simulink model "wheel_leg"  (R2025b)
settings: Solver=VariableStepAuto  StartTime=0.0  StopTime=10  FixedStep=0.0001  RelTol=1e-3
values from neighbouring files (symbols this model uses):
  g = 9.8    [part1_dynamic.m]    (also in simulation.m)
  M_L_support = 1.44/2 + 0.045*2    (= 0.81)    [part1_dynamic.m]
  N = length(x_uniform)    [sweep_Ncut.m]
  N_filter = results(i).N    [sweep_Ncut.m]
  X = [theta; dtheta; x; dx; phi; dphi]    [part1_dynamic.m]    (also in simulation.m)
  Y = fft(x_uniform)    [sweep_Ncut.m]
undefined symbols (not defined in the file or in its folder): KD_leg, KP_leg, Z
libraries: sm_lib x76, nesl_utility x20, slpidlib x4
(part 1 of 3)
settings Model: PauseTimes=10  Creator=Hhop  LastModifiedBy=13422
settings SolverCC: AlgebraicLoopSolver=TrustRegion  MinimalZcImpactIntegration=on
settings DebuggingCC: ReadBeforeWriteMsg=DisableAll  WriteAfterWriteMsg=DisableAll  WriteAfterReadMsg=DisableAll  MultiTaskDSMMsg=none
settings ModelReferenceCC: UpdateModelReferenceTargets=IfOutOfDate
settings SFSimCC: SFSimEcho=off
settings RTWCC: GPUComputeCapability=3.5  DLArmComputeVersion=19.05

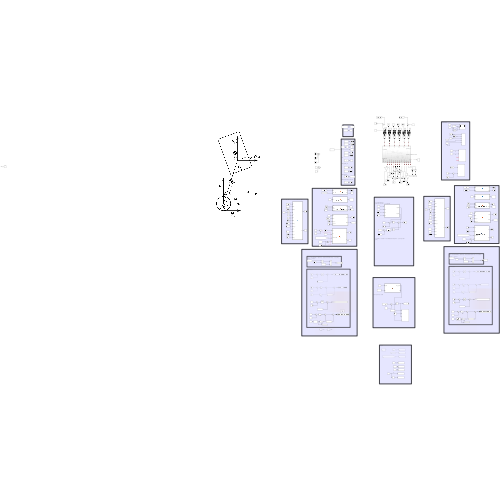
[thumbnail: Simulink's stored preview of the top-level diagram]
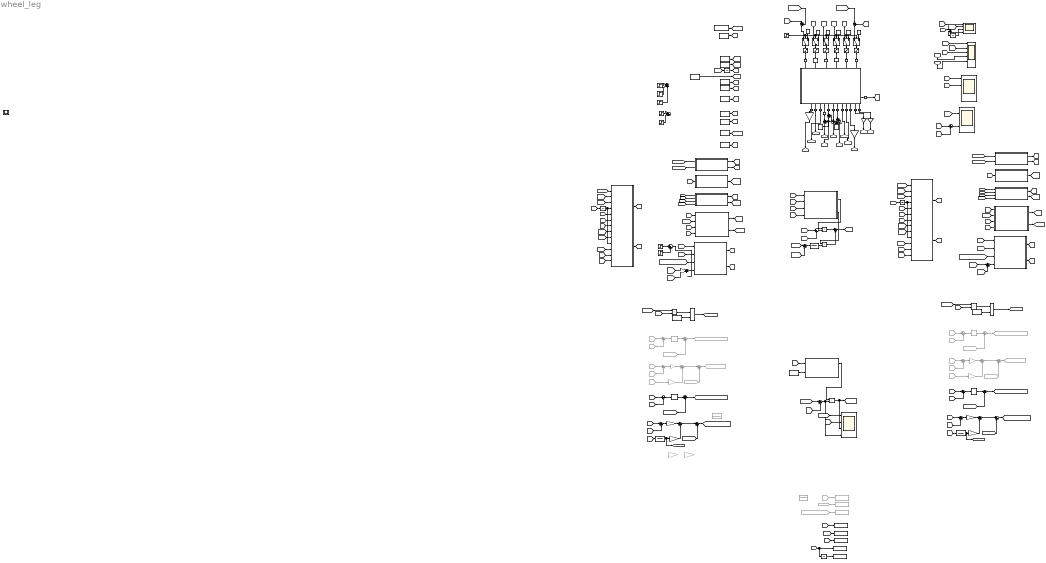
== system wheel_leg ==
  note: 转向控制器
      |
      |
      |
      |
      |
      |
      |
      |
      |
      |
      |
      |
      |
      |
      |
      |
      | 注意从左向右转是正方向啊
  note: 抑制劈叉控制器
      |
      |
      |
      |
      | 这个是等效摆的弹簧阻尼
      | 这个腾空依旧可以控制住，这个是慢控制器
      |
      |
      |
      |
      |
      |
      |
      |
      |
      |
      |
      |
      |
      |
      |
      |
      |
      |
      |
      |
      |
      |
      |
      |
      |
      |
      |
      |
      |
      |
      |
      |
      |
      |
      |
      | 这个是加到轮子上的控制器，在轮子解除地面的时候快速相应，这个是快速控制器
      | (这个和)
  note: 数据实时观测
  note: 数据打印
  note: 整个单边支持力的输出
  note: 腿长保持控制器
  note: 计算单腿支持力前馈，先只用前馈加上去，开环。之后再闭环.
      | 另外，先不除以costheta了，数值不稳定，而且线性化就是大概在1附近。为了更加稳定
      | 直接除以一个衰减因子
  note: X_d
      |
      |
      |
      |
      |
      |
      |
      |
      |
      |
      |
      |
      |
      |
      |
      |
      |
      |
      | L0d
      |
      |
      |
      |
      |
      | pai0_Diff_PD_ctrl
      |
      |
      |
      |
      |
      |
      |
      |
      |
      |
      | yaw轴速度目标
      |
      |
      |
      |
      | yaw轴速度控制器相应速度参数
  note: 这里面dx与x默认RL一样了，之后考虑不对称的时候在改
  note: 整个单边支持力的输出
  note: 腿长保持控制器
  note: 计算单腿支持力前馈，先只用前馈加上去，开环。之后再闭环.
      | 另外，先不除以costheta了，数值不稳定，而且线性化就是大概在1附近。为了更加稳定
      | 直接除以一个衰减因子
  note: 这里面dx与x默认RL一样了，之后考虑不对称的时候在改
  Constant : Constant  Value=M_L_support
  Constant1 : Constant  Value=g
  Constant10 : Constant  Value=1.2
  Constant11 : Constant
  Constant12 : Constant  Value=5
  Constant13 : Constant  Value=0.7
  Constant{2..3,6..7,14..19} (10 alike) : Constant  Value=0
  Constant22 : Constant  Value=0.0603
  Constant23 : Constant  Value=0.5
  Constant24 : Constant  Value=0.5
  Constant4 : Constant  Value=1.2
  Constant5 : Constant  Value=0.08
  Constant8 : Constant  Value=pi/2
  Constant9 : Constant  Value=pi/2
  Divide1 : Product  Inputs=*/
  Divide2 : Product  Inputs=*/
  From{47,52,96,100} (4 alike) : From  Commented=on  GotoTag=L_F_feedforward
  From{48,53,97,101} (4 alike) : From  Commented=on  GotoTag=L0
  From102 : From  Commented=on  GotoTag=dL0
  From{46,51,95,99} (4 alike) : From  Commented=on  GotoTag=L0d
  From54 : From  Commented=on  GotoTag=dL0
  From59 : From  Commented=on  GotoTag=L_F_output_command_jaco_with_filter
  From62 : From  Commented=on  GotoTag=L_dL0
  From67 : From  Commented=on  GotoTag=L_dL0_filterd
  Gain : Gain  Gain=0.0603
  Gain1 : Gain  Gain=-1
  Gain2 : Gain  Gain=-1
  Gain3 : Gain  Gain=0.0603
  Goto28 : Goto  Commented=on  GotoTag=F_output_command_matlab_without_filter
  Goto29 : Goto  Commented=on  GotoTag=F_output_command_jaco
  Goto45 : Goto  Commented=on  GotoTag=F_output_command_matlab_without_filter
  Goto46 : Goto  Commented=on  GotoTag=F_output_command_jaco
  Integrator{,1..4} (5 alike) : Integrator
  KD : Gain  Commented=on  Gain=1000
  KD2 : Gain  Commented=on  Gain=1000
  KD3 : Gain  Commented=on  Gain=KD_leg
  KP : Gain  Commented=on  Gain=220
  KP1 : Gain  Gain=1100
  KP2 : Gain  Commented=on  Gain=220
  KP3 : Gain  Gain=1100
  KP4 : Gain  Gain=31.77
  KP5 : Gain  Commented=on  Gain=KP_leg
  KP6 : Gain  Gain=31.77
  MATLAB Function : MATLAB Function  TreatAsAtomicUnit=on
  MATLAB Function1 : MATLAB Function  TreatAsAtomicUnit=on
  MATLAB Function10 : MATLAB Function  TreatAsAtomicUnit=on
  MATLAB Function11 : MATLAB Function  TreatAsAtomicUnit=on
  MATLAB Function12 : MATLAB Function  TreatAsAtomicUnit=on
  MATLAB Function13 : MATLAB Function  TreatAsAtomicUnit=on
  MATLAB Function2 : MATLAB Function  TreatAsAtomicUnit=on
  MATLAB Function3 : MATLAB Function  TreatAsAtomicUnit=on
  MATLAB Function4 : MATLAB Function  TreatAsAtomicUnit=on
  MATLAB Function5 : MATLAB Function  TreatAsAtomicUnit=on
  MATLAB Function6 : MATLAB Function  TreatAsAtomicUnit=on
  MATLAB Function7 : MATLAB Function  TreatAsAtomicUnit=on
  MATLAB Function8 : MATLAB Function  TreatAsAtomicUnit=on
  MATLAB Function9 : MATLAB Function  TreatAsAtomicUnit=on
  PID Controller : slpidlib/PID Controller  Commented=on  Controller=PID  Form=Parallel  TimeDomain=Continuous-time  UseExternalTs=off  SampleTime=-1  IntegratorMethod=Forward Euler  FilterMethod=Forward Euler  ControllerParametersSource=internal  P=220  I=0  UseKiTs=off  D=1000  UseExternalDerivativeSource=off  N=0  UseFilter=on  TunerSelectOption=Transfer Function Based (PID Tuner App)  InitialConditionSource=internal  InitialConditionForIntegrator=0  InitialConditionForFilter=0  DifferentiatorICPrevScaledInput=0  ExternalReset=none  TrackingMode=off  Kt=1  LimitOutput=off  SatLimitsSource=internal  UpperSaturationLimit=inf  LowerSaturationLimit=-inf  LinearizeAsGain=on  AntiWindupMode=none  Kb=1  LimitIntegrator=off  UpperIntegratorSaturationLimit=inf  LowerIntegratorSaturationLimit=-inf  POutMin=[]  POutMax=[]  IOutMin=[]  IOutMax=[]  DOutMin=[]  DOutMax=[]  NOutMin=[]  NOutMax=[]  SumOutMin=[]  SumOutMax=[]  SaturationOutMin=[]  SaturationOutMax=[]  PParamMin=[]  PParamMax=[]  IParamMin=[]  IParamMax=[]  DParamMin=[]  DParamMax=[]  NParamMin=[]  NParamMax=[]  KbParamMin=[]  KbParamMax=[]  KtParamMin=[]  KtParamMax=[]  KbOutMin=[]  KbOutMax=[]  KtOutMin=[]  KtOutMax=[]  IntegratorOutMin=[]  IntegratorOutMax=[]  FilterOutMin=[]  FilterOutMax=[]  SumI1OutMin=[]  SumI1OutMax=[]  SumI2OutMin=[]  SumI2OutMax=[]  SumI3OutMin=[]  SumI3OutMax=[]  SumI4OutMin=[]  SumI4OutMax=[]  SumDOutMin=[]  SumDOutMax=[]  DifferentiatorOutMin=[]  DifferentiatorOutMax=[]  FilterDiffOutCoefMin=[]  FilterDiffOutCoefMax=[]  ReciprocalOutMin=[]  ReciprocalOutMax=[]  SumDenOutMin=[]  SumDenOutMax=[]  SumNumOutMin=[]  SumNumOutMax=[]  DivideOutMin=[]  DivideOutMax=[]  UdiffTsProdOutMin=[]  UdiffTsProdOutMax=[]  NTsProdOutMin=[]  NTsProdOutMax=[]  UintegralTsProdOutMin=[]  UintegralTsProdOutMax=[]  UngainTsProdOutMin=[]  UngainTsProdOutMax=[]  ClampingZeroOutDataTypeStr=Inherit: Inherit via back propagation  ClampingZeroOutMin=[]  ClampingZeroOutMax=[]  FilterDenConstantOutDataTypeStr=Inherit: Inherit via back propagation  FilterDenConstantOutMin=[]  FilterDenConstantOutMax=[]  PCopyOutDataTypeStr=Inherit: Inherit via back propagation  PCopyOutMin=[]  PCopyOutMax=[]  NCopyOutDataTypeStr=Inherit: Inherit via back propagation  NCopyOutMin=[]  NCopyOutMax=[]  IntegratorContinuousStateAttributes=''  IntegratorStateMustResolveToSignalObject=off  IntegratorRTWStateStorageClass=Auto  FilterContinuousStateAttributes=''  FilterStateMustResolveToSignalObject=off  FilterRTWStateStorageClass=Auto  ParallelPVariant=InternalParameters  IdealPVariant=Disabled  IVariant=InternalParameters  DVariant=InternalParameters  IntegratorVariant=Continuous  SatVariant=Disabled  AWVariant=Passthrough  PCopyVariant=Disabled  TRVariant=Disabled  FdbkBlocksVariant=Forward  IdealPFdbkVariant=Disabled  SatFdbkVariant=Disabled  DerivativeFilterVariant=ContFilter  NVariant=InternalParameters  NCopyVariant=Disabled  FilterICVariant=InternalICsFilter  IntegratorICVariant=InternalICs  ExternalResetVariant=Disabled  TRSumVariant=Passthrough  SumFdbkVariant=Disabled  SumVariant=Sum_PID  TsampFilterVariant=InternalTs  TsampNgainVariant=Passthrough  TsampIntegralVariant=Disabled_SignalSpec  ExternalSaturationOutDataTypeStr=Inherit: Same as second input  DerivativeSourceVariant=ErrorSignal  PreIntVariant=InternalPreInt
  PID Controller1 : slpidlib/PID Controller  Controller=PID  Form=Parallel  TimeDomain=Continuous-time  UseExternalTs=off  SampleTime=-1  IntegratorMethod=Forward Euler  FilterMethod=Forward Euler  ControllerParametersSource=internal  P=220  I=0  UseKiTs=off  D=1000  UseExternalDerivativeSource=off  N=100  UseFilter=on  TunerSelectOption=Transfer Function Based (PID Tuner App)  InitialConditionSource=internal  InitialConditionForIntegrator=0  InitialConditionForFilter=0  DifferentiatorICPrevScaledInput=0  ExternalReset=none  TrackingMode=off  Kt=1  LimitOutput=off  SatLimitsSource=internal  UpperSaturationLimit=inf  LowerSaturationLimit=-inf  LinearizeAsGain=on  AntiWindupMode=none  Kb=1  LimitIntegrator=off  UpperIntegratorSaturationLimit=inf  LowerIntegratorSaturationLimit=-inf  POutMin=[]  POutMax=[]  IOutMin=[]  IOutMax=[]  DOutMin=[]  DOutMax=[]  NOutMin=[]  NOutMax=[]  SumOutMin=[]  SumOutMax=[]  SaturationOutMin=[]  SaturationOutMax=[]  PParamMin=[]  PParamMax=[]  IParamMin=[]  IParamMax=[]  DParamMin=[]  DParamMax=[]  NParamMin=[]  NParamMax=[]  KbParamMin=[]  KbParamMax=[]  KtParamMin=[]  KtParamMax=[]  KbOutMin=[]  KbOutMax=[]  KtOutMin=[]  KtOutMax=[]  IntegratorOutMin=[]  IntegratorOutMax=[]  FilterOutMin=[]  FilterOutMax=[]  SumI1OutMin=[]  SumI1OutMax=[]  SumI2OutMin=[]  SumI2OutMax=[]  SumI3OutMin=[]  SumI3OutMax=[]  SumI4OutMin=[]  SumI4OutMax=[]  SumDOutMin=[]  SumDOutMax=[]  DifferentiatorOutMin=[]  DifferentiatorOutMax=[]  FilterDiffOutCoefMin=[]  FilterDiffOutCoefMax=[]  ReciprocalOutMin=[]  ReciprocalOutMax=[]  SumDenOutMin=[]  SumDenOutMax=[]  SumNumOutMin=[]  SumNumOutMax=[]  DivideOutMin=[]  DivideOutMax=[]  UdiffTsProdOutMin=[]  UdiffTsProdOutMax=[]  NTsProdOutMin=[]  NTsProdOutMax=[]  UintegralTsProdOutMin=[]  UintegralTsProdOutMax=[]  UngainTsProdOutMin=[]  UngainTsProdOutMax=[]  ClampingZeroOutDataTypeStr=Inherit: Inherit via back propagation  ClampingZeroOutMin=[]  ClampingZeroOutMax=[]  FilterDenConstantOutDataTypeStr=Inherit: Inherit via back propagation  FilterDenConstantOutMin=[]  FilterDenConstantOutMax=[]  PCopyOutDataTypeStr=Inherit: Inherit via back propagation  PCopyOutMin=[]  PCopyOutMax=[]  NCopyOutDataTypeStr=Inherit: Inherit via back propagation  NCopyOutMin=[]  NCopyOutMax=[]  IntegratorContinuousStateAttributes=''  IntegratorStateMustResolveToSignalObject=off  IntegratorRTWStateStorageClass=Auto  FilterContinuousStateAttributes=''  FilterStateMustResolveToSignalObject=off  FilterRTWStateStorageClass=Auto  ParallelPVariant=InternalParameters  IdealPVariant=Disabled  IVariant=InternalParameters  DVariant=InternalParameters  IntegratorVariant=Continuous  SatVariant=Disabled  AWVariant=Passthrough  PCopyVariant=Disabled  TRVariant=Disabled  FdbkBlocksVariant=Forward  IdealPFdbkVariant=Disabled  SatFdbkVariant=Disabled  DerivativeFilterVariant=ContFilter  NVariant=InternalParameters  NCopyVariant=Disabled  FilterICVariant=InternalICsFilter  IntegratorICVariant=InternalICs  ExternalResetVariant=Disabled  TRSumVariant=Passthrough  SumFdbkVariant=Disabled  SumVariant=Sum_PID  TsampFilterVariant=InternalTs  TsampNgainVariant=Passthrough  TsampIntegralVariant=Disabled_SignalSpec  ExternalSaturationOutDataTypeStr=Inherit: Same as second input  DerivativeSourceVariant=ErrorSignal  PreIntVariant=InternalPreInt
  PID Controller2 : slpidlib/PID Controller  Commented=on  Controller=PID  Form=Parallel  TimeDomain=Continuous-time  UseExternalTs=off  SampleTime=-1  IntegratorMethod=Forward Euler  FilterMethod=Forward Euler  ControllerParametersSource=internal  P=220  I=0  UseKiTs=off  D=1000  UseExternalDerivativeSource=off  N=0  UseFilter=on  TunerSelectOption=Transfer Function Based (PID Tuner App)  InitialConditionSource=internal  InitialConditionForIntegrator=0  InitialConditionForFilter=0  DifferentiatorICPrevScaledInput=0  ExternalReset=none  TrackingMode=off  Kt=1  LimitOutput=off  SatLimitsSource=internal  UpperSaturationLimit=inf  LowerSaturationLimit=-inf  LinearizeAsGain=on  AntiWindupMode=none  Kb=1  LimitIntegrator=off  UpperIntegratorSaturationLimit=inf  LowerIntegratorSaturationLimit=-inf  POutMin=[]  POutMax=[]  IOutMin=[]  IOutMax=[]  DOutMin=[]  DOutMax=[]  NOutMin=[]  NOutMax=[]  SumOutMin=[]  SumOutMax=[]  SaturationOutMin=[]  SaturationOutMax=[]  PParamMin=[]  PParamMax=[]  IParamMin=[]  IParamMax=[]  DParamMin=[]  DParamMax=[]  NParamMin=[]  NParamMax=[]  KbParamMin=[]  KbParamMax=[]  KtParamMin=[]  KtParamMax=[]  KbOutMin=[]  KbOutMax=[]  KtOutMin=[]  KtOutMax=[]  IntegratorOutMin=[]  IntegratorOutMax=[]  FilterOutMin=[]  FilterOutMax=[]  SumI1OutMin=[]  SumI1OutMax=[]  SumI2OutMin=[]  SumI2OutMax=[]  SumI3OutMin=[]  SumI3OutMax=[]  SumI4OutMin=[]  SumI4OutMax=[]  SumDOutMin=[]  SumDOutMax=[]  DifferentiatorOutMin=[]  DifferentiatorOutMax=[]  FilterDiffOutCoefMin=[]  FilterDiffOutCoefMax=[]  ReciprocalOutMin=[]  ReciprocalOutMax=[]  SumDenOutMin=[]  SumDenOutMax=[]  SumNumOutMin=[]  SumNumOutMax=[]  DivideOutMin=[]  DivideOutMax=[]  UdiffTsProdOutMin=[]  UdiffTsProdOutMax=[]  NTsProdOutMin=[]  NTsProdOutMax=[]  UintegralTsProdOutMin=[]  UintegralTsProdOutMax=[]  UngainTsProdOutMin=[]  UngainTsProdOutMax=[]  ClampingZeroOutDataTypeStr=Inherit: Inherit via back propagation  ClampingZeroOutMin=[]  ClampingZeroOutMax=[]  FilterDenConstantOutDataTypeStr=Inherit: Inherit via back propagation  FilterDenConstantOutMin=[]  FilterDenConstantOutMax=[]  PCopyOutDataTypeStr=Inherit: Inherit via back propagation  PCopyOutMin=[]  PCopyOutMax=[]  NCopyOutDataTypeStr=Inherit: Inherit via back propagation  NCopyOutMin=[]  NCopyOutMax=[]  IntegratorContinuousStateAttributes=''  IntegratorStateMustResolveToSignalObject=off  IntegratorRTWStateStorageClass=Auto  FilterContinuousStateAttributes=''  FilterStateMustResolveToSignalObject=off  FilterRTWStateStorageClass=Auto  ParallelPVariant=InternalParameters  IdealPVariant=Disabled  IVariant=InternalParameters  DVariant=InternalParameters  IntegratorVariant=Continuous  SatVariant=Disabled  AWVariant=Passthrough  PCopyVariant=Disabled  TRVariant=Disabled  FdbkBlocksVariant=Forward  IdealPFdbkVariant=Disabled  SatFdbkVariant=Disabled  DerivativeFilterVariant=ContFilter  NVariant=InternalParameters  NCopyVariant=Disabled  FilterICVariant=InternalICsFilter  IntegratorICVariant=InternalICs  ExternalResetVariant=Disabled  TRSumVariant=Passthrough  SumFdbkVariant=Disabled  SumVariant=Sum_PID  TsampFilterVariant=InternalTs  TsampNgainVariant=Passthrough  TsampIntegralVariant=Disabled_SignalSpec  ExternalSaturationOutDataTypeStr=Inherit: Same as second input  DerivativeSourceVariant=ErrorSignal  PreIntVariant=InternalPreInt
  PID Controller3 : slpidlib/PID Controller  Controller=PID  Form=Parallel  TimeDomain=Continuous-time  UseExternalTs=off  SampleTime=-1  IntegratorMethod=Forward Euler  FilterMethod=Forward Euler  ControllerParametersSource=internal  P=220  I=0  UseKiTs=off  D=1000  UseExternalDerivativeSource=off  N=100  UseFilter=on  TunerSelectOption=Transfer Function Based (PID Tuner App)  InitialConditionSource=internal  InitialConditionForIntegrator=0  InitialConditionForFilter=0  DifferentiatorICPrevScaledInput=0  ExternalReset=none  TrackingMode=off  Kt=1  LimitOutput=off  SatLimitsSource=internal  UpperSaturationLimit=inf  LowerSaturationLimit=-inf  LinearizeAsGain=on  AntiWindupMode=none  Kb=1  LimitIntegrator=off  UpperIntegratorSaturationLimit=inf  LowerIntegratorSaturationLimit=-inf  POutMin=[]  POutMax=[]  IOutMin=[]  IOutMax=[]  DOutMin=[]  DOutMax=[]  NOutMin=[]  NOutMax=[]  SumOutMin=[]  SumOutMax=[]  SaturationOutMin=[]  SaturationOutMax=[]  PParamMin=[]  PParamMax=[]  IParamMin=[]  IParamMax=[]  DParamMin=[]  DParamMax=[]  NParamMin=[]  NParamMax=[]  KbParamMin=[]  KbParamMax=[]  KtParamMin=[]  KtParamMax=[]  KbOutMin=[]  KbOutMax=[]  KtOutMin=[]  KtOutMax=[]  IntegratorOutMin=[]  IntegratorOutMax=[]  FilterOutMin=[]  FilterOutMax=[]  SumI1OutMin=[]  SumI1OutMax=[]  SumI2OutMin=[]  SumI2OutMax=[]  SumI3OutMin=[]  SumI3OutMax=[]  SumI4OutMin=[]  SumI4OutMax=[]  SumDOutMin=[]  SumDOutMax=[]  DifferentiatorOutMin=[]  DifferentiatorOutMax=[]  FilterDiffOutCoefMin=[]  FilterDiffOutCoefMax=[]  ReciprocalOutMin=[]  ReciprocalOutMax=[]  SumDenOutMin=[]  SumDenOutMax=[]  SumNumOutMin=[]  SumNumOutMax=[]  DivideOutMin=[]  DivideOutMax=[]  UdiffTsProdOutMin=[]  UdiffTsProdOutMax=[]  NTsProdOutMin=[]  NTsProdOutMax=[]  UintegralTsProdOutMin=[]  UintegralTsProdOutMax=[]  UngainTsProdOutMin=[]  UngainTsProdOutMax=[]  ClampingZeroOutDataTypeStr=Inherit: Inherit via back propagation  ClampingZeroOutMin=[]  ClampingZeroOutMax=[]  FilterDenConstantOutDataTypeStr=Inherit: Inherit via back propagation  FilterDenConstantOutMin=[]  FilterDenConstantOutMax=[]  PCopyOutDataTypeStr=Inherit: Inherit via back propagation  PCopyOutMin=[]  PCopyOutMax=[]  NCopyOutDataTypeStr=Inherit: Inherit via back propagation  NCopyOutMin=[]  NCopyOutMax=[]  IntegratorContinuousStateAttributes=''  IntegratorStateMustResolveToSignalObject=off  IntegratorRTWStateStorageClass=Auto  FilterContinuousStateAttributes=''  FilterStateMustResolveToSignalObject=off  FilterRTWStateStorageClass=Auto  ParallelPVariant=InternalParameters  IdealPVariant=Disabled  IVariant=InternalParameters  DVariant=InternalParameters  IntegratorVariant=Continuous  SatVariant=Disabled  AWVariant=Passthrough  PCopyVariant=Disabled  TRVariant=Disabled  FdbkBlocksVariant=Forward  IdealPFdbkVariant=Disabled  SatFdbkVariant=Disabled  DerivativeFilterVariant=ContFilter  NVariant=InternalParameters  NCopyVariant=Disabled  FilterICVariant=InternalICsFilter  IntegratorICVariant=InternalICs  ExternalResetVariant=Disabled  TRSumVariant=Passthrough  SumFdbkVariant=Disabled  SumVariant=Sum_PID  TsampFilterVariant=InternalTs  TsampNgainVariant=Passthrough  TsampIntegralVariant=Disabled_SignalSpec  ExternalSaturationOutDataTypeStr=Inherit: Same as second input  DerivativeSourceVariant=ErrorSignal  PreIntVariant=InternalPreInt
  PS-Simulink Converter{,1..11,13} (13 alike) : nesl_utility/PS-Simulink Converter  PhysicalDomain=network_engine_domain  SubClassName=ps_output  LeftPortType=input  RightPortType=output  PseudoPeriodic=off  Frequencies=[]  VectorFormat=inherit  Unit=inherit  AffineConversion=off
  Product{,1..4} (5 alike) : Product
  Saturation : Saturate  UpperLimit=9  LowerLimit=-9
  Saturation{1..4} (4 alike) : Saturate  UpperLimit=100  LowerLimit=-100
  Saturation5 : Saturate  UpperLimit=9  LowerLimit=-9
  Scope : Scope  NumInputPorts=6
      settings: ActiveDisplayYMinimum=-0.39030088912791516  ActiveDisplayYMaximum=1.9087110566025913
  Scope1 : Scope  NumInputPorts=4
      settings: ActiveDisplayYMinimum=-5.5468642131335777  ActiveDisplayYMaximum=4.7288974279093985
  Scope2 : Scope  NumInputPorts=4
      settings: ActiveDisplayYMinimum=0.047567306536691584  ActiveDisplayYMaximum=0.10854014232866921  DataLoggingVariableName=ScopeData2
  Scope3 : Scope  NumInputPorts=2
      settings: ActiveDisplayYMinimum=-9.89781740644245  ActiveDisplayYMaximum=2.6400705173137622  DataLoggingVariableName=ScopeData3
  Scope5 : Scope  NumInputPorts=4
      settings: ActiveDisplayYMinimum=-1.7811758029110956  ActiveDisplayYMaximum=1.308099831593017  DataLoggingVariableName=ScopeData5
  Simulink-PS Converter{,1..5} (6 alike) : nesl_utility/Simulink-PS Converter  PhysicalDomain=network_engine_domain  SubClassName=ps_input  LeftPortType=input  RightPortType=output  PseudoPeriodic=off  Frequencies=[]  NoiseDistribution=none  NoiseParameters=[]  Unit=1  AffineConversion=off  FilteringAndDerivatives=provide  SimscapeFilterOrder=1  InputFilterTimeConstant=0.001  UdotUserProvided=0
  Step : Step  Time=0.2  SampleTime=0
  Step1 : Step  After=-0.3  SampleTime=0
  Step2 : Step  Time=5  After=0.6  SampleTime=0
  Step3 : Step  Time=9  After=-0.3  SampleTime=0
  Step4 : Step  After=-0.3  SampleTime=0
  Step5 : Step  Time=5  After=0.6  SampleTime=0
  Step6 : Step  Time=3.5  After=-3  SampleTime=0
  Step7 : Step  Time=3  After=3  SampleTime=0
  Sum{,1,8,10,13..15,23,27,30,32,34} (12 alike) : Sum  Inputs=|++
  Sum{7,9,11,16,22,24,28..29,31,33} (10 alike) : Sum  Inputs=|+-
  Sum12 : Sum  Inputs=|+++
  Sum{2,4,6,17,19,21} (6 alike) : Sum  Commented=on  Inputs=|+-
  Sum{3,5,18,20} (4 alike) : Sum  Commented=on  Inputs=|++
  Sum25 : Sum  Inputs=|+++
  Sum26 : Sum  Inputs=|+-+
  Sum35 : Sum  Inputs=|-+
  Switch{,1..5} (6 alike) : Switch  Criteria=u2 > Threshold  SaturateOnIntegerOverflow=off  InputSameDT=off
  To Workspace : ToWorkspace  Commented=on  VariableName=F_command_out  SaveFormat=Timeseries  SampleTime=-1
  To Workspace1 : ToWorkspace  VariableName=L0  SaveFormat=Timeseries  SampleTime=-1
  To Workspace2 : ToWorkspace  Commented=on  VariableName=dL0_raw  SaveFormat=Timeseries  SampleTime=-1
  To Workspace3 : ToWorkspace  Commented=on  VariableName=dL0_filterd  SaveFormat=Timeseries  SampleTime=-1
  To Workspace4 : ToWorkspace  VariableName=dxd  SaveFormat=Timeseries  SampleTime=-1
  To Workspace5 : ToWorkspace  VariableName=xd  SaveFormat=Timeseries  SampleTime=-1
  To Workspace8 : ToWorkspace  VariableName=dx  SaveFormat=Timeseries  SampleTime=-1
  To Workspace9 : ToWorkspace  VariableName=x  SaveFormat=Timeseries  SampleTime=-1
  Transfer Fcn1 : TransferFcn  Numerator=[300]  Denominator=[1 300]
  Transfer Fcn2 : TransferFcn  Numerator=[300]  Denominator=[1 300]
  Transfer Fcn3 : TransferFcn  Numerator=[300]  Denominator=[1 300]
  Transfer Fcn4 : TransferFcn  Commented=on  Numerator=[N_filter]  Denominator=[1 N_filter]
  Transfer Fcn5 : TransferFcn  Commented=on  Numerator=[N_filter]  Denominator=[1 N_filter]
  blance_leg_model : Subsystem
      settings: PortSchema="{\"entries\":[{\"content\":{\"sides\":[{\"content\":{\"connectorIds\":[\"LConn1\",\"LConn2\",\"LConn3\",\"LConn4\",\"LConn5\",\"LConn6\"]},\"type\":\"ConnectorPlacement.EquallySpacedRectSide\",\"uuid\":\"df2d0b15-ec70-4430-8d90-67c6d88950b4\"},{\"content\":{\"connectorIds\":[\"RConn1\",\"RConn2\",\"RConn3\",\"RConn4\",\"RConn5\",\"RConn6\",\"RConn7\",\"RConn8\",\"RConn9\",\"RConn10\",\"RConn11\",\"RConn12\",\"RConn13\",\"RConn14\"],\"side\":\"RIGHT\"},\"type\":\"ConnectorPlacement.EquallySpacedRectSide\",\"uuid\":\"ec9b4787-d265-4ad9-b676-e253d2304993\"},{\"content\":{\"connectorIds\":[\"LConn7\",\"LConn8\"],\"side\":\"TOP\"},\"type\":\"ConnectorPlacement.EquallySpacedRectSide\",\"uuid\":\"40dd08fe-dc32-4cee-bbb8-c1ec6d04ee32\"},{\"content\":{\"connectorIds\":[\"RConn15\",\"RConn16\",\"RConn17\"],\"side\":\"BOTTOM\"},\"type\":\"ConnectorPlacement.EquallySpacedRectSide\",\"uuid\":\"0f9c1faf-3e52-4dca-bbb1-0993be9fa88c\"}]},\"type\":\"ConnectorPlacement.EquallySpacedConnector\",\"uuid\":\"d540d646-85aa-4f97-ae4d-1bccec971368\"}],\"packageUris\":[\"http://schema.mathworks.com/mf0/Connector/R2020b\"],\"version\":\"1.0\"}"
  mean_x2 : Scope
      settings: ActiveDisplayYMinimum=-0.05008  ActiveDisplayYMaximum=0.21605  DataLoggingVariableName=ScopeData16
  wires:
  Sum/1 -> [L_pai4]
  PS-Simulink Converter2/1 -> [L_dpai1]
  PS-Simulink Converter1/1 -> [L_dpai4]
  [L_pai4] -> MATLAB Function/2(pai4)
  [L_pai1] -> MATLAB Function/1(pai1)
  MATLAB Function/1(L0) -> [L_L0]
  MATLAB Function/2(pai0) -> [L_pai0]
  [L_L0] -> MATLAB Function1/1(L0)
  MATLAB Function1/1(K) -> [L_K]
  [L_K] -> MATLAB Function2/1(K)
  [L_pai1] -> MATLAB Function3/1(phi1)
  [L_pai4] -> MATLAB Function3/2(phi4)
  [L_dpai1] -> MATLAB Function3/3(dphi1)
  [L_dpai4] -> MATLAB Function3/4(dphi4)
  MATLAB Function3/1(dL0) -> [L_dL0]
  MATLAB Function3/2(dphi0) -> [L_dpai0]
  [L_pai0] -> MATLAB Function4/1(phi0)
  [L_dpai0] -> MATLAB Function4/2(dphi0)
  [pai] -> MATLAB Function4/3(body_phi)
  [dpai] -> MATLAB Function4/4(body_dphi)
  MATLAB Function4/2(dtheta) -> [L_dtheta]
  MATLAB Function4/1(theta) -> [L_theta]
  [L_dtheta] -> MATLAB Function2/3(dtheta)
  [L_dx] -> MATLAB Function2/5(dx)
  [L_dx] -> Integrator/1
  [pai] -> MATLAB Function2/6(phi)
  [dpai] -> MATLAB Function2/7(dphi)
  [L_theta] -> MATLAB Function2/2(theta)
  Constant2/1 -> [theta_d]
  Constant3/1 -> [dtheta_d]
  Integrator1/1 -> [x_d]
  Constant6/1 -> [pai_d]
  Constant7/1 -> [dpai_d]
  [theta_d] -> MATLAB Function2/8(theta_d)
  [dtheta_d] -> MATLAB Function2/9(dtheta_d)
  Integrator/1 -> MATLAB Function2/10(x_d), MATLAB Function2/4(x)
  [dx_d] -> MATLAB Function2/11(dx_d)
  [pai_d] -> MATLAB Function2/12(phi_d)
  [dpai_d] -> MATLAB Function2/13(dphi_d)
  MATLAB Function2/1(T) -> [L_T]
  MATLAB Function2/2(Tp) -> [L_Tp]
  Constant/1 -> [M_L_support]
  Constant1/1 -> [g]
  [M_L_support] -> Product/1
  [g] -> Product/2
  [L_pai1] -> MATLAB Function5/1(phi1)
  [L_pai4] -> MATLAB Function5/2(phi4)
  MATLAB Function5/1(T1) -> [LT1]
  MATLAB Function5/2(T4) -> [LT4]
  PS-Simulink Converter3/1 -> Sum1/1
  Sum1/1 -> [L_pai1]
  PS-Simulink Converter/1 -> Sum/1
  Gain2/1 -> [dpai]
  Saturation2/1 -> Simulink-PS Converter2/1
  Saturation5/1 -> Simulink-PS Converter5/1
  Saturation3/1 -> Simulink-PS Converter3/1
  Sum34/1 -> Switch/1
  Saturation1/1 -> Simulink-PS Converter1/1
  Saturation4/1 -> Simulink-PS Converter4/1
  Saturation/1 -> Simulink-PS Converter/1
  Constant14/1 -> Switch/3
  Switch/1 -> Saturation/1
  Constant15/1 -> Switch1/3
  [LT1] -> Switch1/1
  Constant16/1 -> Switch2/3
  [LT4] -> Switch2/1
  Constant17/1 -> Switch3/3
  [RT4] -> Switch3/1
  Constant18/1 -> Switch4/3
  [RT1] -> Switch4/1
  Constant19/1 -> Switch5/3
  Sum35/1 -> Switch5/1
  Switch1/1 -> Saturation1/1
  Switch2/1 -> Saturation2/1
  Switch3/1 -> Saturation3/1
  Switch4/1 -> Saturation4/1
  Switch5/1 -> Saturation5/1
  Step/1 -> Switch/2, Switch5/2, Switch4/2, Switch3/2, Switch2/2, Switch1/2
  [L_F_output_command_jaco_with_filter] -> MATLAB Function5/3(F_command)
  [dx_d] -> Integrator1/1
  [x_d] -> Scope1/1  "xd"
  [dx_d] -> Scope1/2  "dxd"
  [L_dx] -> Scope1/4, Integrator2/1  "dx"
  Integrator2/1 -> Scope1/3  "x"
  Product/1 -> Divide1/1
  Constant4/1 -> Divide1/2
  Constant5/1 -> [L0d]
  Sum2/1 -> PID Controller/1
  From46/1 -> Sum2/1
  PID Controller/1 -> Sum3/1
  From47/1 -> Sum3/2
  From48/1 -> Sum2/2
  Sum3/1 -> Goto28/1
  [L_L0] -> Scope2/1  "L0"
  [L0d] -> Scope2/2  "L0d"
  Divide1/1 -> [L_F_feedforward]
  From54/1 -> KD/1
  Sum5/1 -> Goto29/1
  KP/1 -> Sum6/1
  Sum4/1 -> KP/1
  Sum6/1 -> Sum5/1
  From53/1 -> Sum4/2
  KD/1 -> Sum6/2
  From52/1 -> Sum5/2
  From51/1 -> Sum4/1
  ? -> Scope2/3
  ? -> Scope2/4
  From59/1 -> To Workspace/1
  [L_L0] -> To Workspace1/1  "L0"
  Sum8/1 -> [L_F_output_command_matlab_with_filter]
  [L_L0] -> Sum7/2
  [L_F_feedforward] -> Sum8/2
  PID Controller1/1 -> Sum8/1
  [L0d] -> Sum7/1
  Sum7/1 -> PID Controller1/1
  From62/1 -> To Workspace2/1  "L0"
  [L0d] -> Sum9/1
  [L_F_feedforward] -> Sum10/2
  KP4/1 -> Sum11/2
  [L_L0] -> Sum9/2
  Sum11/1 -> Sum10/1
  Sum9/1 -> KP3/1
  KP3/1 -> Sum11/1
  Sum10/1 -> [L_F_output_command_jaco_with_filter]
  From67/1 -> To Workspace3/1
  [x_d] -> To Workspace5/1  "xd"
  [dx_d] -> To Workspace4/1  "dxd"
  [L_dx] -> To Workspace8/1, Integrator3/1  "dx"
  Integrator3/1 -> To Workspace9/1  "x"
  PS-Simulink Converter4/1 -> Gain/1
  Gain/1 -> [L_dx]
  [pai] -> Scope/3  "pai"
  [L_pai1] -> Scope/4  "pai1"
  [L_pai4] -> Scope/5  "pai4"
  [L_pai0] -> Scope/2  "pai0"
  [L_theta] -> Scope/1  "theta"
  Constant8/1 -> Sum/2, Sum1/2
  Gain1/1 -> [pai]
  PS-Simulink Converter6/1 -> Gain1/1
  PS-Simulink Converter5/1 -> Gain2/1
  Sum13/1 -> [R_pai1]
  PS-Simulink Converter7/1 -> Sum13/1
  Constant9/1 -> Sum14/2, Sum13/2
  PS-Simulink Converter8/1 -> Sum14/1
  Sum14/1 -> [R_pai4]
  PS-Simulink Converter9/1 -> [R_dpai1]
  PS-Simulink Converter10/1 -> [R_dpai4]
  Sum15/1 -> [R_F_output_command_jaco_with_filter]
  KP1/1 -> Sum16/1
  Sum24/1 -> KP1/1
  Sum16/1 -> Sum15/1
  [R_L0] -> Sum24/2
  KP6/1 -> Sum16/2
  [R_F_feedforward] -> Sum15/2
  [L0d] -> Sum24/1
  Sum22/1 -> PID Controller3/1
  [L0d] -> Sum22/1
  PID Controller3/1 -> Sum23/1
  [L_F_feedforward] -> Sum23/2
  [R_L0] -> Sum22/2
  Sum23/1 -> [R_F_output_command_matlab_with_filter]
  From99/1 -> Sum19/1
  From100/1 -> Sum20/2
  KD2/1 -> Sum21/2
  From101/1 -> Sum19/2
  Sum21/1 -> Sum20/1
  Sum19/1 -> KP2/1
  KP2/1 -> Sum21/1
  Sum20/1 -> Goto46/1
  From102/1 -> KD2/1
  Divide2/1 -> [R_F_feedforward]
  Sum18/1 -> Goto45/1
  From97/1 -> Sum17/2
  From96/1 -> Sum18/2
  PID Controller2/1 -> Sum18/1
  From95/1 -> Sum17/1
  Sum17/1 -> PID Controller2/1
  Constant10/1 -> Divide2/2
  Product1/1 -> Divide2/1
  [R_F_output_command_jaco_with_filter] -> MATLAB Function11/3(F_command)
  MATLAB Function11/2(T4) -> [RT4]
  MATLAB Function11/1(T1) -> [RT1]
  [R_pai4] -> MATLAB Function11/2(phi4)
  [R_pai1] -> MATLAB Function11/1(phi1)
  [g] -> Product1/2
  [M_L_support] -> Product1/1
  MATLAB Function8/2(Tp) -> [R_Tp]
  MATLAB Function8/1(T) -> [R_T]
  [dpai_d] -> MATLAB Function8/13(dphi_d)
  [pai_d] -> MATLAB Function8/12(phi_d)
  [dx_d] -> MATLAB Function8/11(dx_d)
  Integrator4/1 -> MATLAB Function8/10(x_d), MATLAB Function8/4(x)
  [dtheta_d] -> MATLAB Function8/9(dtheta_d)
  [theta_d] -> MATLAB Function8/8(theta_d)
  [R_theta] -> MATLAB Function8/2(theta)
  [dpai] -> MATLAB Function8/7(dphi)
  [pai] -> MATLAB Function8/6(phi)
  [R_dx] -> Integrator4/1
  [R_dx] -> MATLAB Function8/5(dx)
  [R_dtheta] -> MATLAB Function8/3(dtheta)
  MATLAB Function10/1(theta) -> [R_theta]
  MATLAB Function10/2(dtheta) -> [R_dtheta]
  [dpai] -> MATLAB Function10/4(body_dphi)
  [pai] -> MATLAB Function10/3(body_phi)
  [R_dpai0] -> MATLAB Function10/2(dphi0)
  [R_pai0] -> MATLAB Function10/1(phi0)
  MATLAB Function9/2(dphi0) -> [R_dpai0]
  MATLAB Function9/1(dL0) -> [R_dL0]
  [R_dpai4] -> MATLAB Function9/4(dphi4)
  [R_dpai1] -> MATLAB Function9/3(dphi1)
  [R_pai4] -> MATLAB Function9/2(phi4)
  [R_pai1] -> MATLAB Function9/1(phi1)
  [R_K] -> MATLAB Function8/1(K)
  MATLAB Function7/1(K) -> [R_K]
  [R_L0] -> MATLAB Function7/1(L0)
  MATLAB Function6/2(pai0) -> [R_pai0]
  MATLAB Function6/1(L0) -> [R_L0]
  [R_pai4] -> MATLAB Function6/2(pai4)
  PS-Simulink Converter11/1 -> Gain3/1
  [R_pai1] -> MATLAB Function6/1(pai1)
  Gain3/1 -> [R_dx]
  Step1/1 -> Sum12/1
  Step2/1 -> Sum12/2
  Step3/1 -> Sum12/3
  [R_dL0] -> Transfer Fcn1/1
  Step5/1 -> Sum25/2
  Step4/1 -> Sum25/1
  Constant11/1 -> [dx_d]
  [L_dL0] -> Transfer Fcn3/1
  Transfer Fcn3/1 -> KP4/1, [L_dL0_filterd]
  Transfer Fcn1/1 -> KP6/1, [R_dL0_filterd]
  Transfer Fcn2/1 -> Product3/2
  Sum29/1 -> Transfer Fcn2/1
  [L_pai0] -> Sum28/1
  Product3/1 -> Sum27/2
  [R_pai0] -> Sum28/2
  Sum27/1 -> [Tp_diff]
  Sum28/1 -> Product2/2
  Product2/1 -> Sum27/1
  [L_dpai0] -> Sum29/1
  [R_dpai0] -> Sum29/2
  Constant12/1 -> [fn]
  Constant13/1 -> [zeta]
  [fn] -> MATLAB Function12/1(fn)
  [zeta] -> MATLAB Function12/2(zeta)
  [L_L0] -> MATLAB Function12/3(L_L0)
  [R_L0] -> MATLAB Function12/4(R_L0)
  MATLAB Function12/1(KP_theta) -> Product2/1
  MATLAB Function12/2(KD_theta) -> Product3/1
  Sum26/1 -> MATLAB Function5/4(Tp)
  [L_Tp] -> Sum26/1
  [Tp_diff] -> Sum26/2
  [R_Tp] -> Sum30/1
  [Tp_diff] -> Sum30/2
  Sum30/1 -> MATLAB Function11/4(Tp)
  [Tp_diff] -> Scope3/1
  [R_pai0] -> Sum31/2
  [L_pai0] -> Sum31/1
  Sum31/1 -> Scope3/2
  Step6/1 -> Sum32/1
  Step7/1 -> Sum32/2
  Sum32/1 -> ?
  Constant22/1 -> MATLAB Function13/2(r_w)
  Constant24/1 -> [tau]
  [tau] -> MATLAB Function13/1(tau_yaw)
  Constant23/1 -> [yaw_rate_d]
  [yaw_rate_d] -> Sum33/1
  [Z_W] -> Sum33/2
  Sum33/1 -> Scope5/4, Product4/2
  MATLAB Function13/1(KP_yaw_rate) -> Product4/1
  Product4/1 -> [T_yaw_diff], Scope5/3
  [T_yaw_diff] -> Sum34/2
  [L_T] -> Sum34/1
  [R_T] -> Sum35/2
  [T_yaw_diff] -> Sum35/1
  PS-Simulink Converter13/1 -> [Z_W]
  [yaw_rate_d] -> Scope5/1
  [Z_W] -> Scope5/2
  connections:
  blance_leg_model/RConn7 -- PS-Simulink Converter/LConn1
  PS-Simulink Converter1/LConn1 -- blance_leg_model/RConn4
  PS-Simulink Converter2/LConn1 -- blance_leg_model/RConn5
  PS-Simulink Converter4/LConn1 -- blance_leg_model/RConn3
  blance_leg_model/RConn6 -- PS-Simulink Converter3/LConn1
  PS-Simulink Converter5/LConn1 -- blance_leg_model/RConn14
  PS-Simulink Converter6/LConn1 -- blance_leg_model/RConn13
  blance_leg_model/LConn2 -- Simulink-PS Converter1/RConn1
  blance_leg_model/LConn4 -- Simulink-PS Converter3/RConn1
  blance_leg_model/LConn1 -- Simulink-PS Converter/RConn1
  blance_leg_model/LConn3 -- Simulink-PS Converter2/RConn1
  blance_leg_model/LConn5 -- Simulink-PS Converter4/RConn1
  blance_leg_model/LConn6 -- Simulink-PS Converter5/RConn1
  blance_leg_model/RConn8 -- PS-Simulink Converter7/LConn1
  blance_leg_model/RConn9 -- PS-Simulink Converter8/LConn1
  blance_leg_model/RConn10 -- PS-Simulink Converter9/LConn1
  blance_leg_model/RConn11 -- PS-Simulink Converter10/LConn1
  blance_leg_model/RConn12 -- PS-Simulink Converter11/LConn1
  blance_leg_model/RConn17 -- PS-Simulink Converter13/LConn1
